simulink model "sf_superstep"  (R2017b)
settings: Solver=FixedStepDiscrete  StartTime=0.0  StopTime=10.0  FixedStep=1  RelTol=1e-3  EnableMultiTasking=on
settings Model: ExtModeAutoUpdateStatusClock=off  Creator=The MathWorks, Inc.  LastModifiedBy=The MathWorks, Inc.
settings SolverCC: InsertRTBMode=Auto
settings DataIOCC: LimitDataPoints=on  SaveFormat=Array
settings OptimizationCC: ExpressionDepthLimit=2147483647  InitFltsAndDblsToZero=on  LifeSpan=inf
settings DebuggingCC: UnderspecifiedInitializationDetection=Classic  MergeDetectMultiDrivingBlocksExec=none  FcnCallInpInsideContextMsg=warning  StateNameClashWarn=warning  StrictBusMsg=Warning  SFUnexpectedBacktrackingDiag=warning  SFNoUnconditionalDefaultTransitionDiag=warning  SFExecutionAtInitializationDiag=none
settings HardwareCC: ProdBitPerPointer=32  ProdBitPerSizeT=32  ProdBitPerPtrDiffT=32  ProdLargestAtomicFloat=None  ProdIntDivRoundTo=Undefined  ProdEndianess=Unspecified  ProdWordSize=32  ProdHWDeviceType=32-bit Generic
settings ModelReferenceCC: PropagateSignalLabelsOutOfModel=off
settings SFSimCC: SimParseCustomCode=off
settings CodeAppCC: StateflowObjectComments=on
settings GRTTargetCC: TargetLangStandard=C89/C90 (ANSI)  GeneratePreprocessorConditionals=Disable all  CombineOutputUpdateFcns=off  GRTInterface=on
settings ConfigComp: CovMetricSettings=dw  CovHtmlReporting=on  CovSaveCumulativeToWorkspaceVar=on  CovSaveSingleToWorkspaceVar=on  CovExternalEMLEnable=off  CovSFcnEnable=off

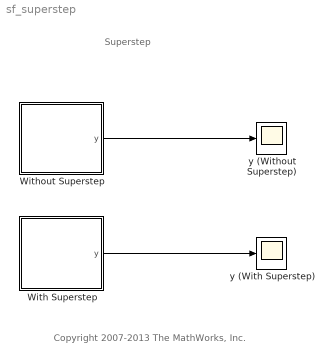
== system sf_superstep ==
  note: Superstep
  note: Copyright 2007-2013 The MathWorks, Inc.
  With Superstep : Stateflow chart  TreatAsAtomicUnit=on
  Without Superstep : Stateflow chart  TreatAsAtomicUnit=on
  y (With Superstep) : Scope
  "y (Without Superstep) " : Scope
  wires:
  Without Superstep/1(y) -> "y (Without Superstep) "/1
  With Superstep/1(y) -> y (With Superstep)/1

== stateflow chart sf_superstep/Without Superstep ==
  state A
    en: y = 1;
  state B
    en: y = 2;
  state C
    en: y = 3;
  (default) -> A : { x = 1; }
  A -> B
  B -> C : [ x == 1 ]
  data: y output double; x local double

== stateflow chart sf_superstep/With Superstep ==
  settings: enableNonTerminalStates=1
  state A
    en: y = 1;
  state B
    en: y = 2;
  state C
    en: y = 3;
  (default) -> A : { x = 1; }
  A -> B
  B -> C : [ x == 1 ]
  data: y output double; x local double
